simulink model "Set_and_Get"  (R2018b)
settings: Solver=FixedStepDiscrete  StartTime=0.0  StopTime=10.0  FixedStep=0.1  RelTol=1e-3
libraries: simulink x7
settings Model: Creator=ZWG  LastModifiedBy=xiaoyang

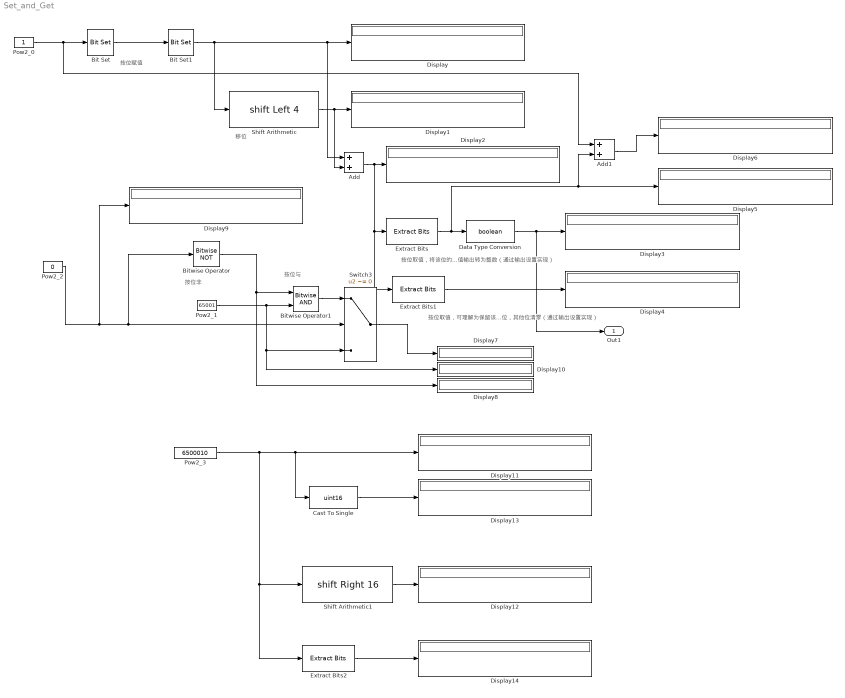
== system Set_and_Get ==
  note: 按位赋值
  note: 移位
  note: 按位取值，将该位的值输出转为整数（通过输出设置实现）
  note: 按位取值，可理解为保留该位，其他位清零（通过输出设置实现）
  note: 按位非
  note: 按位与
  Add : Sum
  Add1 : Sum
  Bit Set : simulink/Logic and Bit Operations/Bit Set  iBit=0
      settings: SourceProductName=Simulink  SourceProductBaseCode=SL
  Bit Set1 : simulink/Logic and Bit Operations/Bit Set  iBit=3
      settings: SourceProductName=Simulink  SourceProductBaseCode=SL
  Bitwise Operator : simulink/Logic and Bit Operations/Bitwise Operator  logicop=NOT  UseBitMask=off  BitMask=bin2dec('11011001')  BitMaskRealWorld=Stored Integer
  Bitwise Operator1 : simulink/Logic and Bit Operations/Bitwise Operator  logicop=AND  UseBitMask=off  NumInputPorts=2  BitMask=bin2dec('11011001')  BitMaskRealWorld=Stored Integer
  Cast To Single : DataTypeConversion  OutDataTypeStr=uint16
  Data Type Conversion : DataTypeConversion  OutDataTypeStr=boolean
  Display{,1..14} (15 alike) : Display
      Display settings: Format=binary (Stored Integer)
      Display1 settings: Format=binary (Stored Integer)
      Display10 settings: Format=binary (Stored Integer)
      Display11 settings: Format=binary (Stored Integer)
      Display12 settings: Format=binary (Stored Integer)
      Display13 settings: Format=binary (Stored Integer)
      Display2 settings: Format=binary (Stored Integer)
      Display7 settings: Format=binary (Stored Integer)
      Display8 settings: Format=binary (Stored Integer)
      Display9 settings: Format=binary (Stored Integer)
  Extract Bits : simulink/Logic and Bit Operations/Extract Bits  bitsToExtract=Range of bits  numBits=8  bitIdxRange=3  outScalingMode=Treat bit field as an integer
      settings: SourceProductName=Simulink
  Extract Bits1 : simulink/Logic and Bit Operations/Extract Bits  bitsToExtract=Range of bits  numBits=8  bitIdxRange=4  outScalingMode=Preserve fixed-point scaling
      settings: SourceProductName=Simulink
  Extract Bits2 : simulink/Logic and Bit Operations/Extract Bits  bitsToExtract=Range of bits  numBits=8  bitIdxRange=0  outScalingMode=Treat bit field as an integer
      settings: SourceProductName=Simulink
  Pow2_0 : Constant  OutDataTypeStr=uint16
  Pow2_1 : Constant  Value=65001  OutDataTypeStr=uint16
  Pow2_2 : Constant  Value=0  OutDataTypeStr=uint16
  Pow2_3 : Constant  Value=6500010  OutDataTypeStr=uint32
  Shift Arithmetic : ArithShift  BitShiftNumber=4  BitShiftDirection=Left
  Shift Arithmetic1 : ArithShift  BitShiftNumber=16  BitShiftDirection=Right
  Switch3 : Switch  Criteria=u2 ~= 0
  Out1 : Outport
  wires:
  Pow2_0/1 -> Add1/1, Bit Set/1
  Bit Set/1 -> Bit Set1/1
  Bit Set1/1 -> Shift Arithmetic/1, Add/1, Display/1
  Shift Arithmetic/1 -> Add/2, Display1/1
  Add/1 -> Extract Bits1/1, Extract Bits/1, Display2/1
  Extract Bits/1 -> Add1/2, Display5/1, Data Type Conversion/1
  Extract Bits1/1 -> Display4/1
  Data Type Conversion/1 -> Out1/1, Display3/1
  Add1/1 -> Display6/1
  Bitwise Operator/1 -> Display8/1, Bitwise Operator1/1
  Pow2_1/1 -> Display10/1, Switch3/3, Bitwise Operator1/2
  Pow2_2/1 -> Display9/1, Bitwise Operator/1, Switch3/2
  Bitwise Operator1/1 -> Switch3/1
  Switch3/1 -> Display7/1
  Pow2_3/1 -> Display11/1, Cast To Single/1, Extract Bits2/1, Shift Arithmetic1/1
  Shift Arithmetic1/1 -> Display12/1
  Cast To Single/1 -> Display13/1
  Extract Bits2/1 -> Display14/1
